simulink model "VCAL_APIS_A_Test_Harness"  (R2023b)
settings: configuration reference "Configuration_Reference" (kept outside this file)
PreLoadFcn:
  | addpath('..\VCAL_Architecture_Demo_Common\');
  | addpath('..\..\VCAL_Architecture_Demo_Common\');
  | 
  | Desktop_Configuration;
InitFcn:
  | create_APIS_A_IO_bus();
settings Model: Creator=IanM  LastModifiedBy=maxju
settings ConfigSetRef: SourceName=Configuration_Reference  SourceLocation=Base Workspace

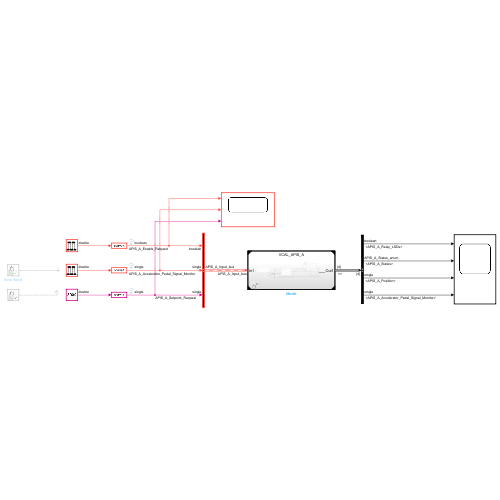
[thumbnail: Simulink's stored preview of the top-level diagram]
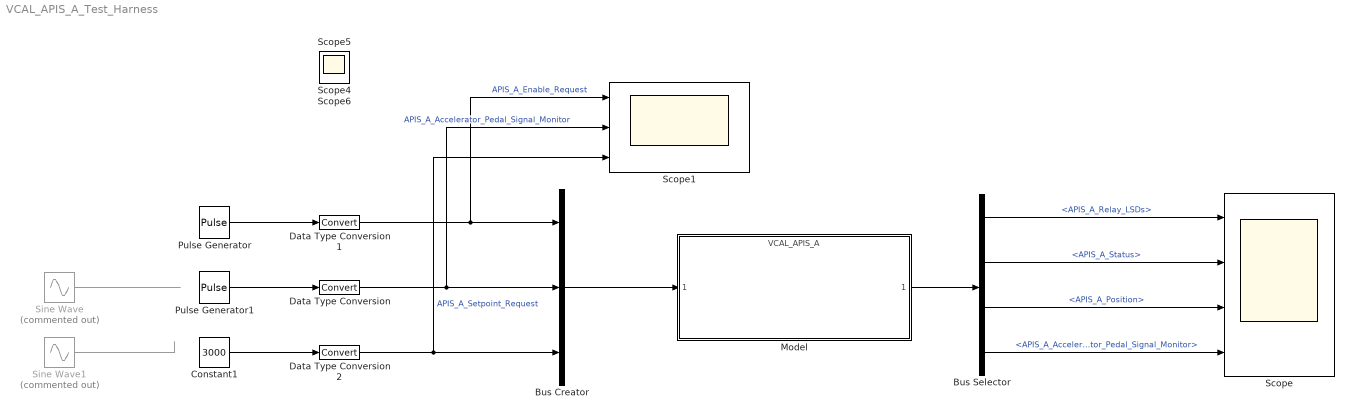
== system VCAL_APIS_A_Test_Harness ==
  Bus Creator : BusCreator  Inputs=3  OutDataTypeStr=Bus: APIS_A_Input_bus  NonVirtualBus=on
      settings: InheritFromInputs=off
  Bus Selector : BusSelector  OutputSignals=APIS_A_Relay_LSDs,APIS_A_Status,APIS_A_Position,APIS_A_Accelerator_Pedal_Signal_Monitor
  Constant1 : Constant  Value=3000
  Data Type Conversion : DataTypeConversion  SaturateOnIntegerOverflow=off  RndMeth=Floor
  Data Type Conversion1 : DataTypeConversion  SaturateOnIntegerOverflow=off  RndMeth=Floor
  Data Type Conversion2 : DataTypeConversion  SaturateOnIntegerOverflow=off  RndMeth=Floor
  Model : ModelReference  ModelNameDialog=VCAL_APIS_A.slx  SimulationMode=Normal  ModelReferenceVersion=1.44
  Pulse Generator : DiscretePulseGenerator  Period=2000  PulseWidth=1000  PhaseDelay=1000  SampleTime=0.001
  Pulse Generator1 : DiscretePulseGenerator  Amplitude=1500  Period=5000  PulseWidth=1500  SampleTime=0.001
  Scope : Scope  NumInputPorts=4
  Scope1 : Scope  NumInputPorts=3
  Sine Wave : Sin  Commented=on  Amplitude=2500  Bias=2500  Frequency=pi  SampleTime=0.001
  Sine Wave1 : Sin  Commented=on  Amplitude=2500  Bias=2500  Frequency=pi  SampleTime=0.001
  Scope4 : Scope
  Scope5 : Scope
  Scope6 : Scope
  wires:
  Model/1 -> Bus Selector/1
  Bus Creator/1 -> Model/1
  Pulse Generator/1 -> Data Type Conversion1/1
  Sine Wave/1 -> ?
  Data Type Conversion/1 -> Scope1/2, Bus Creator/2  "APIS_A_Accelerator_Pedal_Signal_Monitor"
  Sine Wave1/1 -> ?
  Data Type Conversion2/1 -> Scope1/3, Bus Creator/3  "APIS_A_Setpoint_Request"
  Bus Selector/1 -> Scope/1  "<APIS_A_Relay_LSDs>"
  Bus Selector/2 -> Scope/2  "<APIS_A_Status>"
  Bus Selector/3 -> Scope/3  "<APIS_A_Position>"
  Data Type Conversion1/1 -> Scope1/1, Bus Creator/1  "APIS_A_Enable_Request"
  Pulse Generator1/1 -> Data Type Conversion/1
  Constant1/1 -> Data Type Conversion2/1
  Bus Selector/4 -> Scope/4  "<APIS_A_Accelerator_Pedal_Signal_Monitor>"
